simulink model "Simulink_Fourier"  (R2021b)
settings: Solver=VariableStepAuto  StartTime=0.0  StopTime=10.0  RelTol=1e-3
values from neighbouring files (symbols this model uses):
  C = 10    [script - Copiando o exer do professor.m]    (also in script.m)
  fo = 1/T    (= 10)    [script - Copiando o exer do professor.m]    (also in script.m)
  K = 10000    [script - Copiando o exer do professor.m]    (also in script.m)
  M = 1    [script - Copiando o exer do professor.m]    (also in script.m)
settings Model: Creator=55189  LastModifiedBy=55189

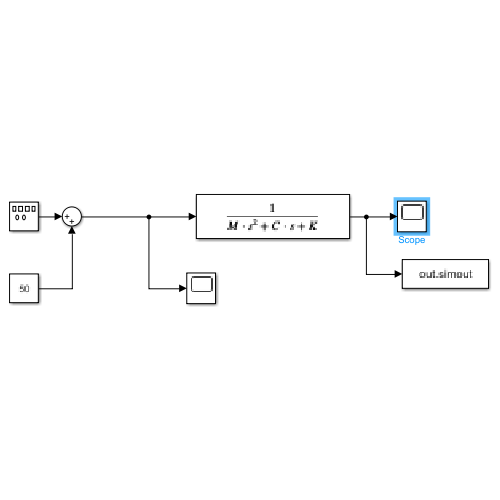
[thumbnail: Simulink's stored preview of the top-level diagram]
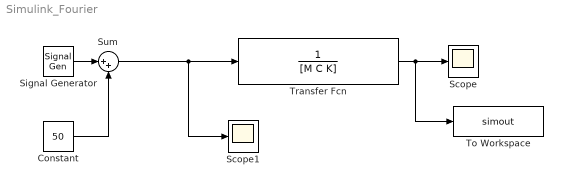
== system Simulink_Fourier ==
  Constant : Constant  Value=50
  Scope : Scope
  Scope1 : Scope
  Signal Generator : SignalGenerator  WaveForm=sawtooth  Amplitude=-50  Frequency=2*pi*fo  Units=rad/sec
  Sum : Sum  Inputs=|++
  To Workspace : ToWorkspace  VariableName=simout  SampleTime=-1
  Transfer Fcn : TransferFcn  Denominator=[M C K]
  wires:
  Signal Generator/1 -> Sum/1
  Transfer Fcn/1 -> To Workspace/1, Scope/1
  Constant/1 -> Sum/2
  Sum/1 -> Scope1/1, Transfer Fcn/1
